simulink model "CoEng_StEng"  (R2016b)
settings: configuration reference "CodeGenConfigSet" (kept outside this file)
values from neighbouring files (symbols this model uses):
  CoEng_nThresCranking_C = Calibration.Parameter    [init_CoEng_StEng.m]    (also in init_CoEng_StEng_SIL.m = Simulink.Parameter)
  CoEng_nThresNrml2Strt_C = Calibration.Parameter    [init_CoEng_StEng.m]    (also in init_CoEng_StEng_SIL.m = Simulink.Parameter)
  CoEng_tiNrml2Strt_C = Calibration.Parameter    [init_CoEng_StEng.m]    (also in init_CoEng_StEng_SIL.m = Simulink.Parameter)
undefined symbols (not defined in the file or in its folder): CoEng_StEng_DT
settings Model: Creator=Colin  LastModifiedBy=zhoutinglin
settings ConfigSetRef: SourceLocation=Base Workspace

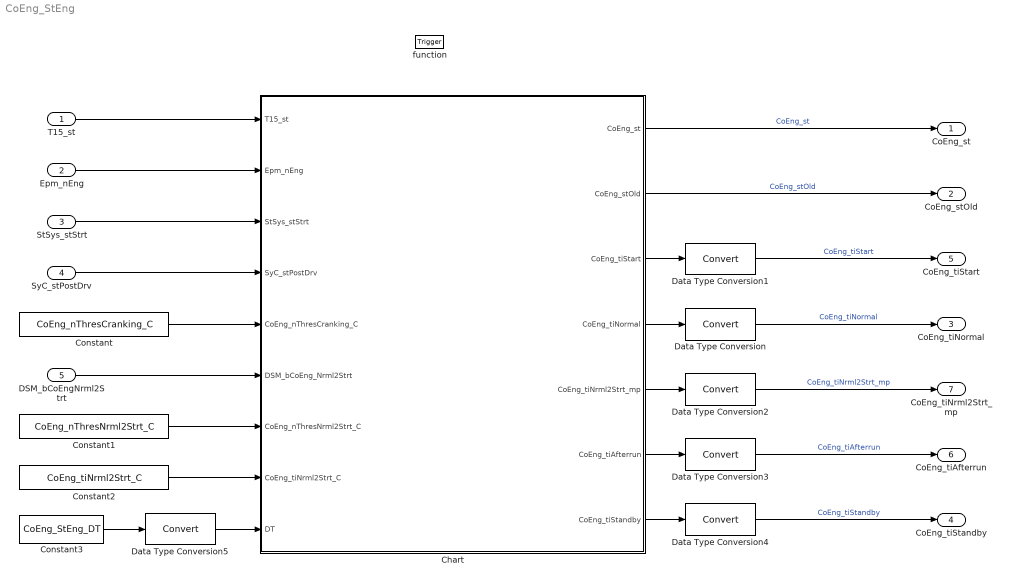
== system CoEng_StEng ==
  T15_st : Inport  Description=Terminal 15 status after debouncing  OutDataTypeStr=Enum: Switch_conv
  Epm_nEng : Inport  Tag=rpm  Description=Engine speed  Port=2  OutMin=0  OutMax=6000  OutDataTypeStr=EngSpeed_rpm
  StSys_stStrt : Inport  Description=state of starting system  Port=3  OutDataTypeStr=Enum: StSys_StrtState_conv
  SyC_stPostDrv : Inport  Description=PostDrive control state  Port=4  OutDataTypeStr=Enum: SyCPostDrvState_conv
  DSM_bCoEngNrml2Strt : Inport  Description=Fault flag to indicate fault inhibit engine start  Port=5  OutMin=0  OutMax=1  OutDataTypeStr=boolean
  function : TriggerPort  TriggerType=function-call  VariantControl=Variant
  Chart : Stateflow chart  TreatAsAtomicUnit=on
  Constant : Constant  Value=CoEng_nThresCranking_C
  Constant1 : Constant  Value=CoEng_nThresNrml2Strt_C
  Constant2 : Constant  Value=CoEng_tiNrml2Strt_C
  Constant3 : Constant  Value=CoEng_StEng_DT  OutMin=1  OutMax=1000
  Data Type Conversion{,1..5} (6 alike) : DataTypeConversion
  CoEng_st : Outport  Description=Engine coordinator state  OutDataTypeStr=Enum: EngState_conv
  CoEng_stOld : Outport  Description=Engine state before current state was reached  Port=2  OutDataTypeStr=Enum: EngState_conv
  CoEng_tiNormal : Outport  Tag=ms  Description="Time since state\"CONENG_RUNNING\"was reached"  Port=3  OutMin=0  OutMax=42949672950  OutDataTypeStr=EngTime_ms
  CoEng_tiStandby : Outport  Tag=ms  Description=Time since engine state COENG_STANDBY was reached  Port=4  OutMin=0  OutMax=42949672950  OutDataTypeStr=EngTime_ms
  CoEng_tiStart : Outport  Tag=ms  Description=Time since state(COENG_READY&COENG_CRANKING) was reached  Port=5  OutMin=0  OutMax=42949672950  OutDataTypeStr=EngTime_ms
  CoEng_tiAfterrun : Outport  Tag=ms  Description=Time since reaching engine state afterrun (COENG-_STOPPING & COENG_FINISH)  Port=6  OutMin=0  OutMax=42949672950  OutDataTypeStr=EngTime_ms
  CoEng_tiNrml2Strt_mp : Outport  Tag=ms  Description=Devounce time for engine state transition from NORMAL to START  Port=7  OutMin=0  OutMax=65535  OutDataTypeStr=EngTime_ms
  wires:
  Chart/1(CoEng_st) -> CoEng_st/1  "CoEng_st"
  Chart/2(CoEng_stOld) -> CoEng_stOld/1  "CoEng_stOld"
  DSM_bCoEngNrml2Strt/1 -> Chart/6(DSM_bCoEng_Nrml2Strt)
  SyC_stPostDrv/1 -> Chart/4(SyC_stPostDrv)
  StSys_stStrt/1 -> Chart/3(StSys_stStrt)
  Epm_nEng/1 -> Chart/2(Epm_nEng)
  T15_st/1 -> Chart/1(T15_st)
  Constant/1 -> Chart/5(CoEng_nThresCranking_C)
  Constant1/1 -> Chart/7(CoEng_nThresNrml2Strt_C)
  Constant2/1 -> Chart/8(CoEng_tiNrml2Strt_C)
  Constant3/1 -> Data Type Conversion5/1
  Chart/3(CoEng_tiStart) -> Data Type Conversion1/1
  Chart/4(CoEng_tiNormal) -> Data Type Conversion/1
  Chart/5(CoEng_tiNrml2Strt_mp) -> Data Type Conversion2/1
  Chart/6(CoEng_tiAfterrun) -> Data Type Conversion3/1
  Chart/7(CoEng_tiStandby) -> Data Type Conversion4/1
  Data Type Conversion/1 -> CoEng_tiNormal/1  "CoEng_tiNormal"
  Data Type Conversion2/1 -> CoEng_tiNrml2Strt_mp/1  "CoEng_tiNrml2Strt_mp"
  Data Type Conversion3/1 -> CoEng_tiAfterrun/1  "CoEng_tiAfterrun"
  Data Type Conversion4/1 -> CoEng_tiStandby/1  "CoEng_tiStandby"
  Data Type Conversion1/1 -> CoEng_tiStart/1  "CoEng_tiStart"
  Data Type Conversion5/1 -> Chart/9(DT)

== stateflow chart CoEng_StEng/Chart ==
  state STANDBY
    entry:
    CoEng_st=EngState_conv.COENG_STANDBY;
    CoEng_stOld=EngState_conv.COENG_STANDBY;
    during:
    CoEng_tiStandby=CoEng_tiStandby+DT;
  state READY
    entry:
    CoEng_stOld=CoEng_st;
    CoEng_st=EngState_conv.COENG_READY;
    during:
    CoEng_tiStart=CoEng_tiStart+DT;
  state FINISH
    entry:
    CoEng_stOld=CoEng_st;
    CoEng_st=EngState_conv.COENG_FINISH;
    during:
    CoEng_tiAfterrun=CoEng_tiAfterrun+DT;
  state STOPPING
    entry:
    CoEng_stOld=CoEng_st;
    CoEng_st=EngState_conv.COENG_STOPPING;
    during:
    CoEng_tiAfterrun=CoEng_tiAfterrun+DT;
  state CRANKING
    entry:
    CoEng_stOld=CoEng_st;
    CoEng_st=EngState_conv.COENG_CRANKING;
    during:
    CoEng_tiStart=CoEng_tiStart+DT;
  state RUNNING
    entry:
    CoEng_stOld=CoEng_st;
    CoEng_st=EngState_conv.COENG_RUNNING;
    CoEng_tiNormal=DT;
    during:
    CoEng_tiNormal=CoEng_tiNormal+DT;
    state TEMP2
      during:CoEng_tiNrml2Strt_mp = CoEng_tiNrml2Strt_mp + DT;
    state TEMP
    state TEMP3
      entry:CoEng_tiNrml2Strt_mp=uint32(0);
    (default) -> TEMP
    TEMP3 -> TEMP2 : [Epm_nEng<CoEng_nThresNrml2Strt_C]
    TEMP2 -> TEMP3 : [Epm_nEng>CoEng_nThresNrml2Strt_C]
    TEMP -> TEMP3
  (default) -> STANDBY
  STANDBY -> READY : [T15_st==1]
  FINISH -> STANDBY [order 1] : [SyC_stPostDrv==8]
  FINISH -> READY [order 2] : [T15_st==1]
  STOPPING -> READY [order 1] : [T15_st==1]
  RUNNING -> READY [order 1] : [(Epm_nEng<CoEng_nThresNrml2Strt_C)&&...
      | (CoEng_tiNrml2Strt_mp>CoEng_tiNrml2Strt_C)&&...
      | (DSM_bCoEng_Nrml2Strt==1)]
  READY -> STOPPING [order 2] : [T15_st==0]
  CRANKING -> READY [order 1] : [Epm_nEng==int16(0)]
  READY -> CRANKING [order 1] : [Epm_nEng>CoEng_nThresCranking_C]
  STOPPING -> FINISH [order 2] : [Epm_nEng==int16(0)]
  CRANKING -> STOPPING [order 3] : [T15_st==0]
  CRANKING -> RUNNING [order 2] : [StSys_stStrt==0]
  RUNNING -> STOPPING [order 2] : [T15_st==0]
  data: T15_st input; Epm_nEng input [0..12799]; StSys_stStrt input; SyC_stPostDrv input; CoEng_st output; CoEng_stOld output; CoEng_nThresCranking_C input [0..12799]; DSM_bCoEng_Nrml2Strt input [0..1]; CoEng_nThresNrml2Strt_C input [0..12799]; CoEng_tiNrml2Strt_C input [0..65535]; DT input uint32; CoEng_tiStart output uint32 size=1 =uint32(0); CoEng_tiNormal output uint32 size=1 =uint32(0); CoEng_tiNrml2Strt_mp output uint32 size=1 [0..65535] =uint32(0); CoEng_tiAfterrun output uint32 size=1 =uint32(0); CoEng_tiStandby output uint32 size=1 =uint32(0)
